simulink model "Grid_Search_control_model"  (R2019a)
settings: Solver=VariableStepAuto  StartTime=0.0  StopTime=0.2  MaxStep=0.001  RelTol=1e-3
values from neighbouring files (symbols this model uses):
  TF11 = tfest(data1,2,1)    [TFEXTRACT.m]
  TF12 = tfest(data1,2,2)    [TFEXTRACT.m]
  TF2 = tfest(data1,3,1)    [TFEXTRACT.m]
  TF3 = tfest(data1,3,2)    [TFEXTRACT.m]
libraries: simulink x1
settings Model: Creator=DELL  LastModifiedBy=DELL

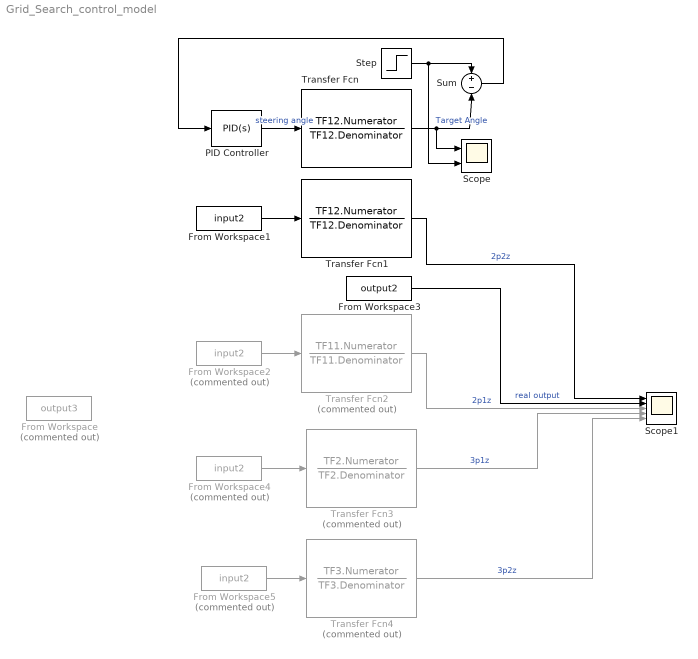
== system Grid_Search_control_model ==
  From Workspace : FromWorkspace  Commented=on  VariableName=output3  SampleTime=0
  From Workspace1 : FromWorkspace  VariableName=input2  SampleTime=0
  From Workspace2 : FromWorkspace  Commented=on  VariableName=input2  SampleTime=0
  From Workspace3 : FromWorkspace  VariableName=output2  SampleTime=0
  From Workspace4 : FromWorkspace  Commented=on  VariableName=input2  SampleTime=0
  From Workspace5 : FromWorkspace  Commented=on  VariableName=input2  SampleTime=0
  PID Controller : simulink/Continuous/PID Controller  Controller=PID  Form=Parallel  TimeDomain=Continuous-time  SampleTime=-1  IntegratorMethod=Forward Euler  FilterMethod=Forward Euler  ControllerParametersSource=internal  P=5.5  I=550  D=0.012  UseFilter=on  N=2200  TunerSelectOption=Transfer Function Based (PID Tuner App)  InitialConditionSource=internal  InitialConditionForIntegrator=0  InitialConditionForFilter=0  DifferentiatorICPrevScaledInput=0  ExternalReset=none  TrackingMode=off  Kt=1  LimitOutput=off  UpperSaturationLimit=inf  LowerSaturationLimit=-inf  LinearizeAsGain=on  AntiWindupMode=none  Kb=1  POutMin=[]  POutMax=[]  IOutMin=[]  IOutMax=[]  DOutMin=[]  DOutMax=[]  NOutMin=[]  NOutMax=[]  SumOutMin=[]  SumOutMax=[]  SaturationOutMin=[]  SaturationOutMax=[]  PParamMin=[]  PParamMax=[]  IParamMin=[]  IParamMax=[]  DParamMin=[]  DParamMax=[]  NParamMin=[]  NParamMax=[]  KbParamMin=[]  KbParamMax=[]  KtParamMin=[]  KtParamMax=[]  KbOutMin=[]  KbOutMax=[]  KtOutMin=[]  KtOutMax=[]  IntegratorOutMin=[]  IntegratorOutMax=[]  FilterOutMin=[]  FilterOutMax=[]  SumI1OutMin=[]  SumI1OutMax=[]  SumI2OutMin=[]  SumI2OutMax=[]  SumI3OutMin=[]  SumI3OutMax=[]  SumI4OutMin=[]  SumI4OutMax=[]  SumDOutMin=[]  SumDOutMax=[]  DifferentiatorOutMin=[]  DifferentiatorOutMax=[]  FilterDiffOutCoefMin=[]  FilterDiffOutCoefMax=[]  ReciprocalOutMin=[]  ReciprocalOutMax=[]  SumDenOutMin=[]  SumDenOutMax=[]  SumNumOutMin=[]  SumNumOutMax=[]  DivideOutMin=[]  DivideOutMax=[]  IntegratorContinuousStateAttributes=''  IntegratorStateMustResolveToSignalObject=off  IntegratorRTWStateStorageClass=Auto  FilterContinuousStateAttributes=''  FilterStateMustResolveToSignalObject=off  FilterRTWStateStorageClass=Auto  ParallelPVariant=InternalParameters  IdealPVariant=Disabled  IVariant=InternalParameters  DVariant=InternalParameters  IntegratorVariant=Continuous  SatVariant=Disabled  AWVariant=Passthrough  PCopyVariant=Disabled  TRVariant=Disabled  FdbkBlocksVariant=Forward  IdealPFdbkVariant=Disabled  SatFdbkVariant=Disabled  DerivativeFilterVariant=ContFilter  NVariant=InternalParameters  NCopyVariant=Disabled  FilterICVariant=InternalICsFilter  IntegratorICVariant=InternalICs  ExternalResetVariant=Disabled  TRSumVariant=Passthrough  SumFdbkVariant=Disabled  SumVariant=Sum_PID
  Scope : Scope  NumInputPorts=2
  Scope1 : Scope  NumInputPorts=5
  Step : Step  Time=0  SampleTime=0
  Sum : Sum  Inputs=+-
  Transfer Fcn : TransferFcn  Numerator=TF12.Numerator  Denominator=TF12.Denominator
  Transfer Fcn1 : TransferFcn  Numerator=TF12.Numerator  Denominator=TF12.Denominator
  Transfer Fcn2 : TransferFcn  Commented=on  Numerator=TF11.Numerator  Denominator=TF11.Denominator
  Transfer Fcn3 : TransferFcn  Commented=on  Numerator=TF2.Numerator  Denominator=TF2.Denominator
  Transfer Fcn4 : TransferFcn  Commented=on  Numerator=TF3.Numerator  Denominator=TF3.Denominator
  wires:
  Transfer Fcn2/1 -> Scope1/3  "2p1z"
  From Workspace3/1 -> Scope1/2  "real output"
  PID Controller/1 -> Transfer Fcn/1  "steering angle"
  From Workspace2/1 -> Transfer Fcn2/1
  Transfer Fcn/1 -> Sum/2, Scope/1  "Target Angle"
  From Workspace1/1 -> Transfer Fcn1/1
  Transfer Fcn1/1 -> Scope1/1  "2p2z"
  Sum/1 -> PID Controller/1
  Step/1 -> Scope/2, Sum/1
  From Workspace4/1 -> Transfer Fcn3/1
  From Workspace5/1 -> Transfer Fcn4/1
  Transfer Fcn3/1 -> Scope1/4  "3p1z"
  Transfer Fcn4/1 -> Scope1/5  "3p2z"
